simulink model "Simulador_Teclado"  (R2015a)
settings: Solver=ode45  StartTime=0.0  StopTime=Inf  MaxStep=1  RelTol=1e-3
StopFcn:
  | close all
  | post_simulacion
model workspace (MAT data in the model file):
  m = 3.797
  b = 2.1
  c = 0.3571
  Salar = 0.75
  AR = 5.88
  cg = [0.44 0 0]
  Ix = 1.229
  Iy = 0.1702
  Iz = 0.8808
  Ixz = 0.9343
  e = 0.9935
  alpha0 = 0.267
  coefprop = [0.016415 -0.0142726]
  C_L0 = 0.0254
  C_Lalpha = 4.0191
  C_Lq = 3.8954
  C_Ldelta_e = 0.5872
  C_D0 = 0.0102
  C_Dbeta1 = -2.0864e-07
  C_Dbeta2 = 0.0671
  C_Dq = 0
  C_Ddelta_e = 0.8461
  C_Y0 = 3.2049e-18
  C_Ybeta = -0.1949
  C_Yp = -0.1172
  C_Yr = 0.0959
  C_Ydelta_a = -0.0696
  C_l0 = 1.1518e-18
  C_lbeta = -0.0765
  C_lp = -0.4018
  C_lr = 0.025
  C_ldelta_a = 0.2987
  C_m0 = 0.018
  C_malpha = -0.2524
  C_mq = -1.3047
  C_mdelta_e = -0.4857
  C_n0 = -2.2667e-07
  C_nbeta = 0.0403
  C_np = -0.0247
  C_nr = -0.1252
  C_ndelta_a = 0.0076
  gamma = 0.20958671
  gamma1 = 8.64638926772
  gamma2 = 7.15127867602
  gamma3 = 4.20255654569
  gamma4 = 4.4578208227
  gamma5 = -2.04582843713
  gamma6 = 5.48942420682
  gamma7 = 10.3736620037
  gamma8 = 5.86392142899
  C_p0 = -1.01045424588e-06
  C_pbeta = -0.14184539659
  C_pp = -1.79869539438
  C_pr = -0.45305525336
  C_pdelta_a = 1.28918307845
  C_r0 = -1.3291750703e-06
  C_rbeta = -0.104707259349
  C_rp = -1.93599126586
  C_rr = -0.622717442342
  C_rdelta_a = 1.3761168826
  C_mp = -0.2168
values from neighbouring files (symbols this model uses):
  r = [r_n;r_e;r_d]    [segmento.m]
  waypoints = reshape(waypoints_mat.',[],1)    [plan_de_vuelo.m]
undefined symbols (not defined in the file or in its folder): F, Light, magnitude, MIL, plan_de_vuelo
libraries: aerolibconvert2 x18, simulink_extras x10, aerolibfltsims x2, simulink x2, instrumentlib x1, aerolibatmos2 x1, aerolibtransform2 x1, aerolibwind2 x1, aerolibgravity2 x1
(part 3 of 3)

== system Simulador_Teclado/Entrada de control manual/Reconocedor de teclado/Subsistema de accion del interruptor de eventos8 ==
  Pulsacion : Inport  PortDimensions=1
  Puerto de accion : ActionPort  ActionType=case
  Boton_ : Outport
  wires:
  Pulsacion/1 -> Boton_/1

== system Simulador_Teclado/Entrada de control manual/Reconocedor de teclado/Subsistema de accion del interruptor de eventos9 ==
  Pulsacion : Inport  PortDimensions=1
  Puerto de accion : ActionPort  ActionType=case
  Boton_ : Outport
  wires:
  Pulsacion/1 -> Boton_/1

== system Simulador_Teclado/Mision/Gestor de GPS/Envio de datos ==
  Datos : Inport
  Activador : EnablePort
  Envio mediante protocolo UDP : instrumentlib/UDP Send  Host=localhost  Port=3333  LocalPort=3334  EnableBlockingMode=on  ByteOrder=BigEndian
  wires:
  Datos/1 -> Envio mediante protocolo UDP/1

== system Simulador_Teclado/Mision/Reconocedor de reinicio de FMS/Posicion_NED de reinicio ==
  Posicion_NED : Inport
  Disparador : TriggerPort  StatesWhenEnabling=reset  ShowOutputPort=on  PortDimensions=1
  Interruptor : Switch  Criteria=u2 > Threshold
  Tierra : Ground
  Posicion_NED_ : Outport
  wires:
  Posicion_NED/1 -> Interruptor/1
  Interruptor/1 -> Posicion_NED_/1
  Disparador/1 -> Interruptor/2
  Tierra/1 -> Interruptor/3
